simulink subsystem "TWFG"  (R2021a)
settings: Solver=VariableStepAuto  StartTime=0.0  StopTime=10.0  RelTol=1e-3
libraries: simulink x2, simulink_extras x1
settings Model: Creator=oscar  LastModifiedBy=oscar

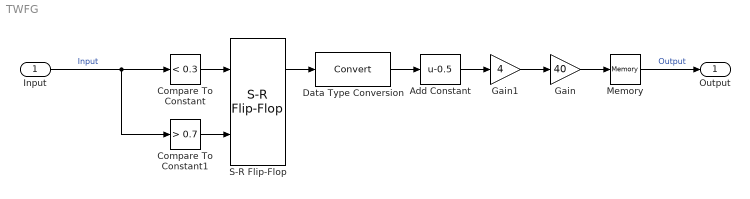
== system TWFG ==
  Input : Inport
  Add Constant : Bias  Bias=-0.5
  Compare To Constant : simulink/Logic and Bit Operations/Compare To Constant  relop=<  const=0.3  OutDataTypeStr=boolean
  Compare To Constant1 : simulink/Logic and Bit Operations/Compare To Constant  relop=>  const=0.7  OutDataTypeStr=boolean
  Data Type Conversion : DataTypeConversion
  Gain : Gain  Gain=40
  Gain1 : Gain  Gain=4
  Memory : Memory
  S-R Flip-Flop : simulink_extras/Flip Flops/S-R Flip-Flop  initial_condition=0
  Output : Outport
  wires:
  Input/1 -> Compare To Constant/1, Compare To Constant1/1  "Input"
  Data Type Conversion/1 -> Add Constant/1
  Compare To Constant1/1 -> S-R Flip-Flop/2
  Gain/1 -> Memory/1
  Add Constant/1 -> Gain1/1
  Compare To Constant/1 -> S-R Flip-Flop/1
  S-R Flip-Flop/1 -> Data Type Conversion/1
  Memory/1 -> Output/1  "Output"
  Gain1/1 -> Gain/1
